simulink library "autolibbatterycommon"  (R2019b)
settings: Solver=ode45  StartTime=0.0  StopTime=10.0  RelTol=1e-3  EnableMultiTasking=on
undefined symbols (not defined in the file or in its folder): BattCap, BattCapInit, BattChargeMax, BattTempBp, C, C1, C2, C3, C4, C5, Cap_LUT, CapacityAh, CapLUTBp, CapSOCBp, CapVolt, Current_BP, DiscIntNeverNeededParam, Em, InitialCapVoltage, InitialChargeRemAh, Np, Ns, R, R0, R1, R2, R3, R4, R5, RefBlkName, RInt, SOC_BP, T1, Tc, Temp_BP, Temperature_BP, Ts, Vinit, Vu
libraries: $bdroot x72, autolibpowerinfoutils x1
(part 1 of 2)
settings Model: ModifiedByFormat=The MathWorks, Inc.  Creator=The MathWorks, Inc.  LastModifiedBy=The MathWorks, Inc.
settings DataIOCC: LimitDataPoints=on  SaveFormat=Array  ReturnWorkspaceOutputs=off
settings OptimizationCC: LifeSpan=inf
settings DebuggingCC: AllowSymbolicDim=off  PregeneratedLibrarySubsystemCodeDiagnostic=none  SFUnexpectedBacktrackingDiag=warning  SFNoUnconditionalDefaultTransitionDiag=warning  SFExecutionAtInitializationDiag=none  ArithmeticOperatorsInVariantConditions=warning
settings HardwareCC: ProdBitPerPointer=32  ProdBitPerSizeT=32  ProdBitPerPtrDiffT=32  ProdLargestAtomicFloat=None  ProdIntDivRoundTo=Undefined  ProdEndianess=Unspecified  ProdWordSize=32  ProdHWDeviceType=32-bit Generic
settings ModelReferenceCC: PropagateSignalLabelsOutOfModel=off
settings SFSimCC: SimUseLocalCustomCode=off  CustomCodeUndefinedFunction=UseInterfaceOnly
settings RTWCC: RTWUseLocalCustomCode=off
settings CodeAppCC: StateflowObjectComments=on
settings GRTTargetCC: TargetLangStandard=C89/C90 (ANSI)  GeneratePreprocessorConditionals=Disable all
settings ConfigComp: CovMetricSettings=dw  CovHtmlReporting=on  CovSaveCumulativeToWorkspaceVar=on  CovSaveSingleToWorkspaceVar=on  CovShowResultsExplorer=off  CovExternalEMLEnable=off

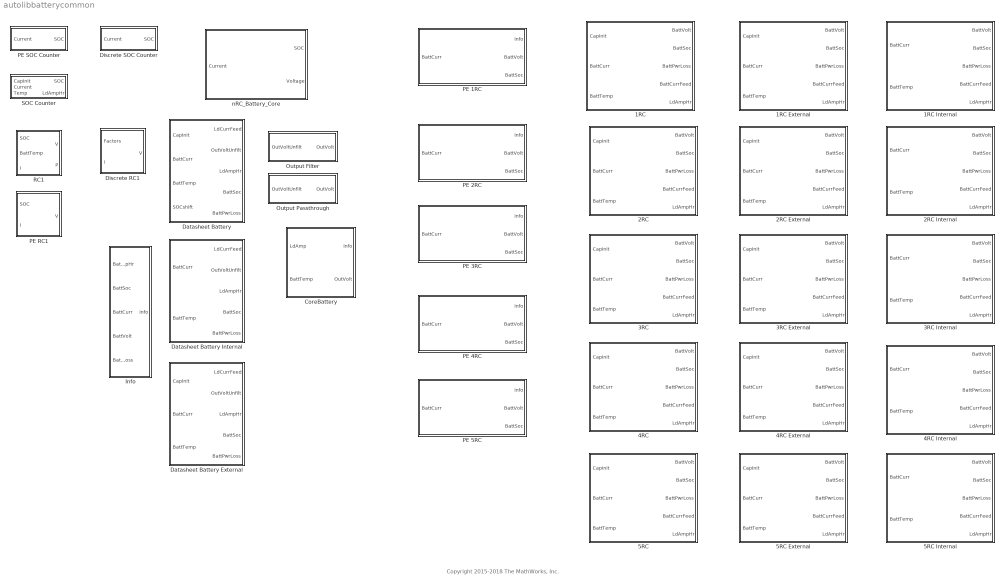
== system autolibbatterycommon ==
  note: Copyright 2015-2018 The MathWorks, Inc.
  1RC : Subsystem  VariantControl=1
  1RC External : Subsystem
  1RC Internal : Subsystem
  2RC : Subsystem  VariantControl=1
  2RC External : Subsystem
  2RC Internal : Subsystem
  3RC : Subsystem  VariantControl=1
  3RC External : Subsystem
  3RC Internal : Subsystem
  4RC : Subsystem  VariantControl=1
  4RC External : Subsystem
  4RC Internal : Subsystem
  5RC : Subsystem  VariantControl=1
  5RC External : Subsystem
  5RC Internal : Subsystem
  CoreBattery : Subsystem
  Datasheet Battery : Subsystem
  Datasheet Battery External : Subsystem
  Datasheet Battery Internal : Subsystem
  Discrete RC1 : Subsystem  mask(RCBlock){R=R1, Tau=T1, SOC_LUT=SOC_BP, Current_BP=Current_BP, V_init=InitialCapVoltage(1), V_upper=Vu(1), V_lower=Vu(1), T=Ts}
      mask prompts: R "Parallel Resistance Lookup Table"; Tau "Parallel Time Constant Lookup Table"; SOC_LUT "SOC Breakpoints"; Current_BP "Current Breakpoints"; V_init "Initial Voltage Across Capacitor"; V_upper "Upper Integrator Voltage Limit"; V_lower "Lower Integrator Voltage Limit"; T "Sample Time"
      mask help: Models a resistor and capacitor in parallel. Both components may vary with SOC.
  Discrete SOC Counter : Subsystem  mask(AhCounter){Q_init=InitialChargeRemAh, Cap=CapacityAh, T=Ts}
      mask prompts: Q_init "Initial Charge (Q)"; Cap "Capacity (Ah)"; T "Sample Time (s)"
      mask help: This is a system that keeps track of SOC by counting coulombs.
  Info : Subsystem  mask{RefBlkName=RefBlkName}
      mask prompts: RefBlkName "Reference block name:"
      mask TypeOptions RefBlkName: Power Accounting Bus Creator/RefBlkName
  Output Filter : Subsystem
  Output Passthrough : Subsystem
  PE 1RC : Subsystem  VariantControl=1
  PE 2RC : Subsystem  VariantControl=2
  PE 3RC : Subsystem  VariantControl=3
  PE 4RC : Subsystem  VariantControl=4
  PE 5RC : Subsystem  VariantControl=5
  PE RC1 : Subsystem  mask(RCBlock){R=R, C=C, SOC_BP=SOC_BP, V_init=CapVolt, V_upper=Inf, V_lower=-Inf}
      mask prompts: R "Parallel Resistance Lookup Table"; C "Parallel Capacitance Lookup Table"; SOC_BP "SOC Breakpoints"; V_init "Initial Voltage Across Capacitor"; V_upper "Upper Integrator Voltage Limit"; V_lower "Lower Integrator Voltage Limit"
      mask help: Models a resistor and capacitor in parallel. Both components may vary with SOC.
  PE SOC Counter : Subsystem  mask(AhCounter){Q_init=BattCapInit, Cap=BattCap}
      mask prompts: Q_init "Initial Charge"; Cap "Capacity"
      mask help: This is a system that keeps track of SOC by counting coulombs.
  RC1 : Subsystem  mask(RCBlock){R=R, C=C, SOC_BP=SOC_BP, Temperature_BP=Temp_BP, V_init=CapVolt, V_upper=Inf, V_lower=-Inf}
      mask prompts: R "Parallel Resistance Lookup Table"; C "Parallel Capacitance Lookup Table"; SOC_BP "SOC Breakpoints"; Temperature_BP "Temperature Breakpoints"; V_init "Initial Voltage Across Capacitor"; V_upper "Upper Integrator Voltage Limit"; V_lower "Lower Integrator Voltage Limit"
      mask help: Models a resistor and capacitor in parallel. Both components may vary with SOC.
  SOC Counter : Subsystem  mask(AhCounter){Q_init=BattCapInit, Cap=BattCap, Cap_LUT=Cap_LUT, Temp_BP=Temperature_BP}
      mask prompts: Q_init "Initial Charge"; Cap "Capacity"; Cap_LUT "Capacity temperature table"; Temp_BP "Temperature Break Points"
      mask help: This is a system that keeps track of SOC by counting coulombs.
  nRC_Battery_Core : Subsystem  VariantControlMode=Label  Variant=on  LabelModeActiveChoice=3

== system autolibbatterycommon/1RC ==
  CapInit : Inport  Unit=A*hr
  BattCurr : Inport  Port=2  Unit=A
  BattTemp : Inport  Port=3  Unit=K
  Em : Lookup_n-D  LookupTableObject=''  BreakpointsForDimension1=SOC_BP  BreakpointsForDimension2=Temperature_BP  Table=Em  ExtrapMethod=Clip  UseLastTableValue=on  InternalRulePriority=Speed  RndMeth=Simplest  InputSameDT=on
  Power : Subsystem
  R0 : Lookup_n-D  LookupTableObject=''  BreakpointsForDimension1=SOC_BP  BreakpointsForDimension2=Temperature_BP  Table=R0  ExtrapMethod=Clip  UseLastTableValue=on  InternalRulePriority=Speed  RndMeth=Simplest  InputSameDT=on
  RC1 : $bdroot/RC1  R=R1  C=C1  SOC_BP=SOC_BP  Temperature_BP=Temperature_BP  V_init=InitialCapVoltage(1)  V_upper=Vu  V_lower=Vl
  SOC Counter : $bdroot/SOC Counter  Q_init=BattCapInit  Cap=BattCap  Cap_LUT=BattCap  Temp_BP=Temperature_BP
  Voltage : Subsystem
  BattVolt : Outport  Unit=V  VectorParamsAs1DForOutWhenUnconnected=off
  BattSoc : Outport  Port=2  Unit=1  VectorParamsAs1DForOutWhenUnconnected=off
  BattPwrLoss : Outport  Port=3  Unit=W  VectorParamsAs1DForOutWhenUnconnected=off
  BattCurrFeed : Outport  Port=4  Unit=A  VectorParamsAs1DForOutWhenUnconnected=off
  LdAmpHr : Outport  Port=5  Unit=A*h  VectorParamsAs1DForOutWhenUnconnected=off
  wires:
  SOC Counter/1 -> R0/1, RC1/1, Em/1, BattSoc/1
  BattCurr/1 -> SOC Counter/2, Power/2(BattAmp), Voltage/3(BattAmp), BattCurrFeed/1, RC1/3
  BattTemp/1 -> SOC Counter/3, RC1/2, R0/2, Em/2
  Em/1 -> Voltage/1(Em)
  R0/1 -> Power/1(R0), Voltage/2(R0)
  RC1/1 -> Voltage/4(RC1)
  Voltage/1(BattVolt) -> BattVolt/1
  Power/1(BattPwrLoss) -> BattPwrLoss/1
  RC1/2 -> Power/3(P1)
  CapInit/1 -> SOC Counter/1
  SOC Counter/2 -> LdAmpHr/1

== system autolibbatterycommon/1RC External ==
  CapInit : Inport
  BattCurr : Inport  Port=2
  BattTemp : Inport  Port=3
  1RC : $bdroot/1RC  SystemSampleTime=-1  VariantControl=1  Latency=0  AutoFrameSizeCalculation=off
  BattVolt : Outport  VectorParamsAs1DForOutWhenUnconnected=off
  BattSoc : Outport  Port=2  VectorParamsAs1DForOutWhenUnconnected=off
  BattPwrLoss : Outport  Port=3  VectorParamsAs1DForOutWhenUnconnected=off
  BattCurrFeed : Outport  Port=4  VectorParamsAs1DForOutWhenUnconnected=off
  LdAmpHr : Outport  Port=5  VectorParamsAs1DForOutWhenUnconnected=off
  wires:
  BattCurr/1 -> 1RC/2
  BattTemp/1 -> 1RC/3
  1RC/1 -> BattVolt/1
  1RC/2 -> BattSoc/1
  1RC/3 -> BattPwrLoss/1
  1RC/4 -> BattCurrFeed/1
  CapInit/1 -> 1RC/1
  1RC/5 -> LdAmpHr/1

== system autolibbatterycommon/1RC Internal ==
  BattCurr : Inport
  BattTemp : Inport  Port=2
  1RC : $bdroot/1RC  SystemSampleTime=-1  VariantControl=1  Latency=0  AutoFrameSizeCalculation=off
  Constant1 : Constant  Value=BattCapInit
  BattVolt : Outport  VectorParamsAs1DForOutWhenUnconnected=off
  BattSoc : Outport  Port=2  VectorParamsAs1DForOutWhenUnconnected=off
  BattPwrLoss : Outport  Port=3  VectorParamsAs1DForOutWhenUnconnected=off
  BattCurrFeed : Outport  Port=4  VectorParamsAs1DForOutWhenUnconnected=off
  LdAmpHr : Outport  Port=5  VectorParamsAs1DForOutWhenUnconnected=off
  wires:
  BattCurr/1 -> 1RC/2
  BattTemp/1 -> 1RC/3
  1RC/1 -> BattVolt/1
  1RC/2 -> BattSoc/1
  1RC/3 -> BattPwrLoss/1
  1RC/4 -> BattCurrFeed/1
  Constant1/1 -> 1RC/1
  1RC/5 -> LdAmpHr/1

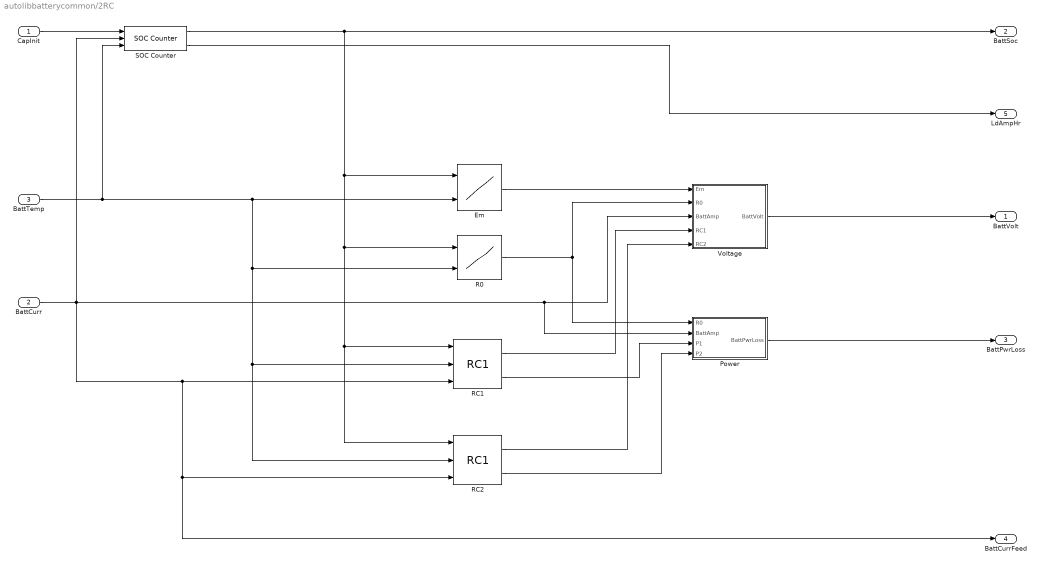
== system autolibbatterycommon/2RC ==
  CapInit : Inport  Unit=A*hr
  BattCurr : Inport  Port=2  Unit=A
  BattTemp : Inport  Port=3  Unit=K
  Em : Lookup_n-D  LookupTableObject=''  BreakpointsForDimension1=SOC_BP  BreakpointsForDimension2=Temperature_BP  Table=Em  ExtrapMethod=Clip  UseLastTableValue=on  InternalRulePriority=Speed  RndMeth=Simplest  InputSameDT=on
  Power : Subsystem
  R0 : Lookup_n-D  LookupTableObject=''  BreakpointsForDimension1=SOC_BP  BreakpointsForDimension2=Temperature_BP  Table=R0  ExtrapMethod=Clip  UseLastTableValue=on  InternalRulePriority=Speed  RndMeth=Simplest  InputSameDT=on
  RC1 : $bdroot/RC1  R=R1  C=C1  SOC_BP=SOC_BP  Temperature_BP=Temperature_BP  V_init=InitialCapVoltage(1)  V_upper=Vu  V_lower=Vl
  RC2 : $bdroot/RC1  R=R2  C=C2  SOC_BP=SOC_BP  Temperature_BP=Temperature_BP  V_init=InitialCapVoltage(2)  V_upper=Vu  V_lower=Vl
  SOC Counter : $bdroot/SOC Counter  Q_init=BattCapInit  Cap=BattCap  Cap_LUT=BattCap  Temp_BP=Temperature_BP
  Voltage : Subsystem
  BattVolt : Outport  Unit=V  VectorParamsAs1DForOutWhenUnconnected=off
  BattSoc : Outport  Port=2  Unit=1  VectorParamsAs1DForOutWhenUnconnected=off
  BattPwrLoss : Outport  Port=3  Unit=W  VectorParamsAs1DForOutWhenUnconnected=off
  BattCurrFeed : Outport  Port=4  Unit=A  VectorParamsAs1DForOutWhenUnconnected=off
  LdAmpHr : Outport  Port=5  Unit=A*h  VectorParamsAs1DForOutWhenUnconnected=off
  wires:
  SOC Counter/1 -> R0/1, RC2/1, RC1/1, Em/1, BattSoc/1
  BattCurr/1 -> SOC Counter/2, Power/2(BattAmp), Voltage/3(BattAmp), BattCurrFeed/1, RC2/3, RC1/3
  BattTemp/1 -> SOC Counter/3, RC2/2, RC1/2, R0/2, Em/2
  Em/1 -> Voltage/1(Em)
  R0/1 -> Power/1(R0), Voltage/2(R0)
  RC1/1 -> Voltage/4(RC1)
  RC2/1 -> Voltage/5(RC2)
  Voltage/1(BattVolt) -> BattVolt/1
  RC1/2 -> Power/3(P1)
  RC2/2 -> Power/4(P2)
  Power/1(BattPwrLoss) -> BattPwrLoss/1
  CapInit/1 -> SOC Counter/1
  SOC Counter/2 -> LdAmpHr/1

== system autolibbatterycommon/2RC External ==
  CapInit : Inport
  BattCurr : Inport  Port=2
  BattTemp : Inport  Port=3
  2RC : $bdroot/2RC  SystemSampleTime=-1  VariantControl=1  Latency=0  AutoFrameSizeCalculation=off
  BattVolt : Outport  VectorParamsAs1DForOutWhenUnconnected=off
  BattSoc : Outport  Port=2  VectorParamsAs1DForOutWhenUnconnected=off
  BattPwrLoss : Outport  Port=3  VectorParamsAs1DForOutWhenUnconnected=off
  BattCurrFeed : Outport  Port=4  VectorParamsAs1DForOutWhenUnconnected=off
  LdAmpHr : Outport  Port=5  VectorParamsAs1DForOutWhenUnconnected=off
  wires:
  BattTemp/1 -> 2RC/3
  BattCurr/1 -> 2RC/2
  CapInit/1 -> 2RC/1
  2RC/1 -> BattVolt/1
  2RC/2 -> BattSoc/1
  2RC/3 -> BattPwrLoss/1
  2RC/4 -> BattCurrFeed/1
  2RC/5 -> LdAmpHr/1

== system autolibbatterycommon/2RC Internal ==
  BattCurr : Inport
  BattTemp : Inport  Port=2
  2RC : $bdroot/2RC  SystemSampleTime=-1  VariantControl=1  Latency=0  AutoFrameSizeCalculation=off
  Constant1 : Constant  Value=BattCapInit
  BattVolt : Outport  VectorParamsAs1DForOutWhenUnconnected=off
  BattSoc : Outport  Port=2  VectorParamsAs1DForOutWhenUnconnected=off
  BattPwrLoss : Outport  Port=3  VectorParamsAs1DForOutWhenUnconnected=off
  BattCurrFeed : Outport  Port=4  VectorParamsAs1DForOutWhenUnconnected=off
  LdAmpHr : Outport  Port=5  VectorParamsAs1DForOutWhenUnconnected=off
  wires:
  BattTemp/1 -> 2RC/3
  BattCurr/1 -> 2RC/2
  2RC/1 -> BattVolt/1
  2RC/2 -> BattSoc/1
  2RC/3 -> BattPwrLoss/1
  2RC/4 -> BattCurrFeed/1
  Constant1/1 -> 2RC/1
  2RC/5 -> LdAmpHr/1

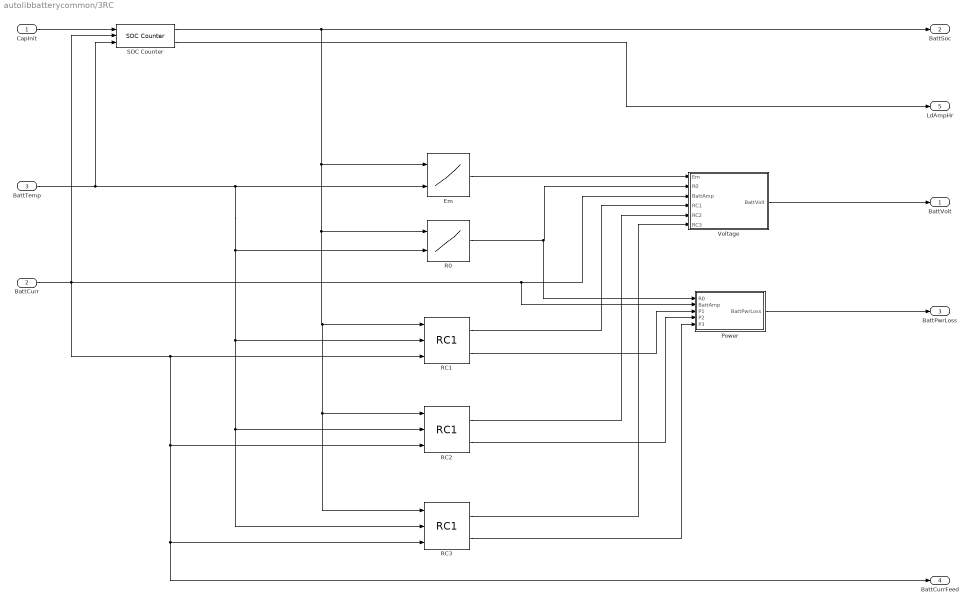
== system autolibbatterycommon/3RC ==
  CapInit : Inport  Unit=A*hr
  BattCurr : Inport  Port=2  Unit=A
  BattTemp : Inport  Port=3  Unit=K
  Em : Lookup_n-D  LookupTableObject=''  BreakpointsForDimension1=SOC_BP  BreakpointsForDimension2=Temperature_BP  Table=Em  ExtrapMethod=Clip  UseLastTableValue=on  InternalRulePriority=Speed  RndMeth=Simplest  InputSameDT=on
  Power : Subsystem
  R0 : Lookup_n-D  LookupTableObject=''  BreakpointsForDimension1=SOC_BP  BreakpointsForDimension2=Temperature_BP  Table=R0  ExtrapMethod=Clip  UseLastTableValue=on  InternalRulePriority=Speed  RndMeth=Simplest  InputSameDT=on
  RC1 : $bdroot/RC1  R=R1  C=C1  SOC_BP=SOC_BP  Temperature_BP=Temperature_BP  V_init=InitialCapVoltage(1)  V_upper=Vu  V_lower=Vl
  RC2 : $bdroot/RC1  R=R2  C=C2  SOC_BP=SOC_BP  Temperature_BP=Temperature_BP  V_init=InitialCapVoltage(2)  V_upper=Vu  V_lower=Vl
  RC3 : $bdroot/RC1  R=R3  C=C3  SOC_BP=SOC_BP  Temperature_BP=Temperature_BP  V_init=InitialCapVoltage(3)  V_upper=Vu  V_lower=Vl
  SOC Counter : $bdroot/SOC Counter  Q_init=BattCapInit  Cap=BattCap  Cap_LUT=BattCap  Temp_BP=Temperature_BP
  Voltage : Subsystem
  BattVolt : Outport  Unit=V  VectorParamsAs1DForOutWhenUnconnected=off
  BattSoc : Outport  Port=2  Unit=1  VectorParamsAs1DForOutWhenUnconnected=off
  BattPwrLoss : Outport  Port=3  Unit=W  VectorParamsAs1DForOutWhenUnconnected=off
  BattCurrFeed : Outport  Port=4  Unit=A  VectorParamsAs1DForOutWhenUnconnected=off
  LdAmpHr : Outport  Port=5  Unit=A*h  VectorParamsAs1DForOutWhenUnconnected=off
  wires:
  BattTemp/1 -> SOC Counter/3, Em/2, R0/2, RC1/2, RC3/2, RC2/2
  BattCurr/1 -> SOC Counter/2, Power/2(BattAmp), Voltage/3(BattAmp), RC1/3, RC2/3, BattCurrFeed/1, RC3/3
  SOC Counter/1 -> Em/1, RC1/1, RC3/1, RC2/1, R0/1, BattSoc/1
  Em/1 -> Voltage/1(Em)
  R0/1 -> Power/1(R0), Voltage/2(R0)
  RC1/1 -> Voltage/4(RC1)
  RC2/1 -> Voltage/5(RC2)
  RC3/1 -> Voltage/6(RC3)
  Voltage/1(BattVolt) -> BattVolt/1
  RC1/2 -> Power/3(P1)
  RC2/2 -> Power/4(P2)
  RC3/2 -> Power/5(P3)
  Power/1(BattPwrLoss) -> BattPwrLoss/1
  CapInit/1 -> SOC Counter/1
  SOC Counter/2 -> LdAmpHr/1

== system autolibbatterycommon/3RC External ==
  CapInit : Inport
  BattCurr : Inport  Port=2
  BattTemp : Inport  Port=3
  3RC : $bdroot/3RC  SystemSampleTime=-1  VariantControl=1  Latency=0  AutoFrameSizeCalculation=off
  BattVolt : Outport  VectorParamsAs1DForOutWhenUnconnected=off
  BattSoc : Outport  Port=2  VectorParamsAs1DForOutWhenUnconnected=off
  BattPwrLoss : Outport  Port=3  VectorParamsAs1DForOutWhenUnconnected=off
  BattCurrFeed : Outport  Port=4  VectorParamsAs1DForOutWhenUnconnected=off
  LdAmpHr : Outport  Port=5  VectorParamsAs1DForOutWhenUnconnected=off
  wires:
  3RC/4 -> BattCurrFeed/1
  3RC/2 -> BattSoc/1
  3RC/1 -> BattVolt/1
  3RC/3 -> BattPwrLoss/1
  BattTemp/1 -> 3RC/3
  BattCurr/1 -> 3RC/2
  CapInit/1 -> 3RC/1
  3RC/5 -> LdAmpHr/1

== system autolibbatterycommon/3RC Internal ==
  BattCurr : Inport
  BattTemp : Inport  Port=2
  3RC : $bdroot/3RC  SystemSampleTime=-1  VariantControl=1  Latency=0  AutoFrameSizeCalculation=off
  Constant1 : Constant  Value=BattCapInit
  BattVolt : Outport  VectorParamsAs1DForOutWhenUnconnected=off
  BattSoc : Outport  Port=2  VectorParamsAs1DForOutWhenUnconnected=off
  BattPwrLoss : Outport  Port=3  VectorParamsAs1DForOutWhenUnconnected=off
  BattCurrFeed : Outport  Port=4  VectorParamsAs1DForOutWhenUnconnected=off
  LdAmpHr : Outport  Port=5  VectorParamsAs1DForOutWhenUnconnected=off
  wires:
  3RC/4 -> BattCurrFeed/1
  3RC/2 -> BattSoc/1
  3RC/1 -> BattVolt/1
  3RC/3 -> BattPwrLoss/1
  BattTemp/1 -> 3RC/3
  BattCurr/1 -> 3RC/2
  Constant1/1 -> 3RC/1
  3RC/5 -> LdAmpHr/1

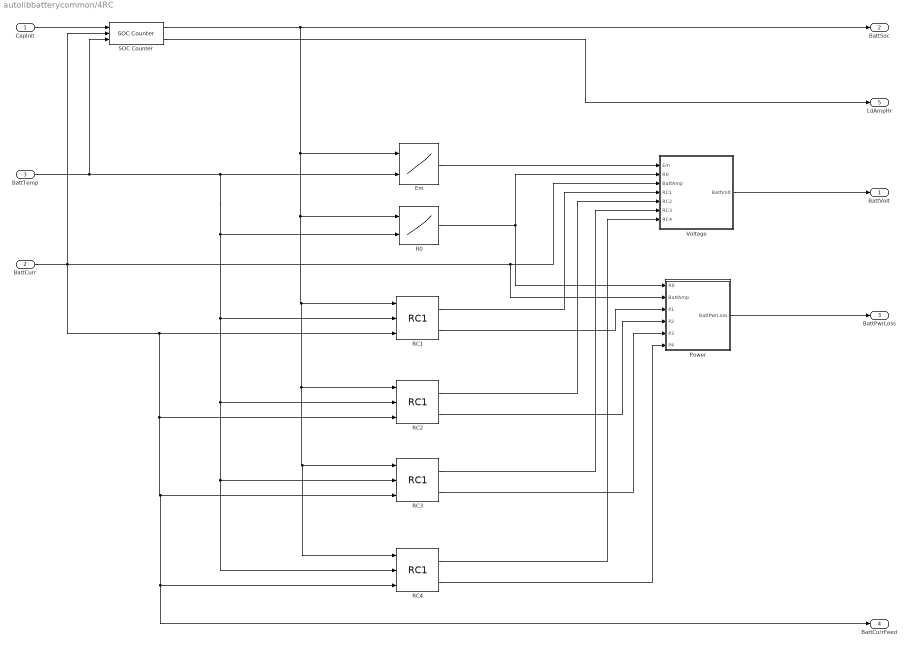
== system autolibbatterycommon/4RC ==
  CapInit : Inport  Unit=A*hr
  BattCurr : Inport  Port=2  Unit=A
  BattTemp : Inport  Port=3  Unit=K
  Em : Lookup_n-D  LookupTableObject=''  BreakpointsForDimension1=SOC_BP  BreakpointsForDimension2=Temperature_BP  Table=Em  ExtrapMethod=Clip  UseLastTableValue=on  InternalRulePriority=Speed  RndMeth=Simplest  InputSameDT=on
  Power : Subsystem
  R0 : Lookup_n-D  LookupTableObject=''  BreakpointsForDimension1=SOC_BP  BreakpointsForDimension2=Temperature_BP  Table=R0  ExtrapMethod=Clip  UseLastTableValue=on  InternalRulePriority=Speed  RndMeth=Simplest  InputSameDT=on
  RC1 : $bdroot/RC1  R=R1  C=C1  SOC_BP=SOC_BP  Temperature_BP=Temperature_BP  V_init=InitialCapVoltage(1)  V_upper=Vu  V_lower=Vl
  RC2 : $bdroot/RC1  R=R2  C=C2  SOC_BP=SOC_BP  Temperature_BP=Temperature_BP  V_init=InitialCapVoltage(2)  V_upper=Vu  V_lower=Vl
  RC3 : $bdroot/RC1  R=R3  C=C3  SOC_BP=SOC_BP  Temperature_BP=Temperature_BP  V_init=InitialCapVoltage(3)  V_upper=Vu  V_lower=Vl
  RC4 : $bdroot/RC1  R=R4  C=C4  SOC_BP=SOC_BP  Temperature_BP=Temperature_BP  V_init=InitialCapVoltage(4)  V_upper=Vu  V_lower=Vl
  SOC Counter : $bdroot/SOC Counter  Q_init=BattCapInit  Cap=BattCap  Cap_LUT=BattCap  Temp_BP=Temperature_BP
  Voltage : Subsystem
  BattVolt : Outport  Unit=V  VectorParamsAs1DForOutWhenUnconnected=off
  BattSoc : Outport  Port=2  Unit=1  VectorParamsAs1DForOutWhenUnconnected=off
  BattPwrLoss : Outport  Port=3  Unit=W  VectorParamsAs1DForOutWhenUnconnected=off
  BattCurrFeed : Outport  Port=4  Unit=A  VectorParamsAs1DForOutWhenUnconnected=off
  LdAmpHr : Outport  Port=5  Unit=A*h  VectorParamsAs1DForOutWhenUnconnected=off
  wires:
  SOC Counter/1 -> R0/1, RC2/1, RC4/1, RC3/1, RC1/1, Em/1, BattSoc/1
  BattCurr/1 -> SOC Counter/2, Power/2(BattAmp), Voltage/3(BattAmp), RC4/3, BattCurrFeed/1, RC3/3, RC2/3, RC1/3
  BattTemp/1 -> SOC Counter/3, RC2/2, RC4/2, RC3/2, RC1/2, R0/2, Em/2
  Em/1 -> Voltage/1(Em)
  R0/1 -> Power/1(R0), Voltage/2(R0)
  RC1/1 -> Voltage/4(RC1)
  RC2/1 -> Voltage/5(RC2)
  RC3/1 -> Voltage/6(RC3)
  RC4/1 -> Voltage/7(RC4)
  Voltage/1(BattVolt) -> BattVolt/1
  Power/1(BattPwrLoss) -> BattPwrLoss/1
  RC1/2 -> Power/3(P1)
  RC2/2 -> Power/4(P2)
  RC3/2 -> Power/5(P3)
  RC4/2 -> Power/6(P4)
  CapInit/1 -> SOC Counter/1
  SOC Counter/2 -> LdAmpHr/1

== system autolibbatterycommon/4RC External ==
  CapInit : Inport
  BattCurr : Inport  Port=2
  BattTemp : Inport  Port=3
  4RC : $bdroot/4RC  SystemSampleTime=-1  VariantControl=1  Latency=0  AutoFrameSizeCalculation=off
  BattVolt : Outport  VectorParamsAs1DForOutWhenUnconnected=off
  BattSoc : Outport  Port=2  VectorParamsAs1DForOutWhenUnconnected=off
  BattPwrLoss : Outport  Port=3  VectorParamsAs1DForOutWhenUnconnected=off
  BattCurrFeed : Outport  Port=4  VectorParamsAs1DForOutWhenUnconnected=off
  LdAmpHr : Outport  Port=5  VectorParamsAs1DForOutWhenUnconnected=off
  wires:
  BattTemp/1 -> 4RC/3
  BattCurr/1 -> 4RC/2
  CapInit/1 -> 4RC/1
  4RC/1 -> BattVolt/1
  4RC/2 -> BattSoc/1
  4RC/3 -> BattPwrLoss/1
  4RC/4 -> BattCurrFeed/1
  4RC/5 -> LdAmpHr/1

== system autolibbatterycommon/4RC Internal ==
  BattCurr : Inport
  BattTemp : Inport  Port=2
  4RC : $bdroot/4RC  SystemSampleTime=-1  VariantControl=1  Latency=0  AutoFrameSizeCalculation=off
  Constant1 : Constant  Value=BattCapInit
  BattVolt : Outport  VectorParamsAs1DForOutWhenUnconnected=off
  BattSoc : Outport  Port=2  VectorParamsAs1DForOutWhenUnconnected=off
  BattPwrLoss : Outport  Port=3  VectorParamsAs1DForOutWhenUnconnected=off
  BattCurrFeed : Outport  Port=4  VectorParamsAs1DForOutWhenUnconnected=off
  LdAmpHr : Outport  Port=5  VectorParamsAs1DForOutWhenUnconnected=off
  wires:
  BattTemp/1 -> 4RC/3
  BattCurr/1 -> 4RC/2
  4RC/1 -> BattVolt/1
  4RC/2 -> BattSoc/1
  4RC/3 -> BattPwrLoss/1
  4RC/4 -> BattCurrFeed/1
  Constant1/1 -> 4RC/1
  4RC/5 -> LdAmpHr/1

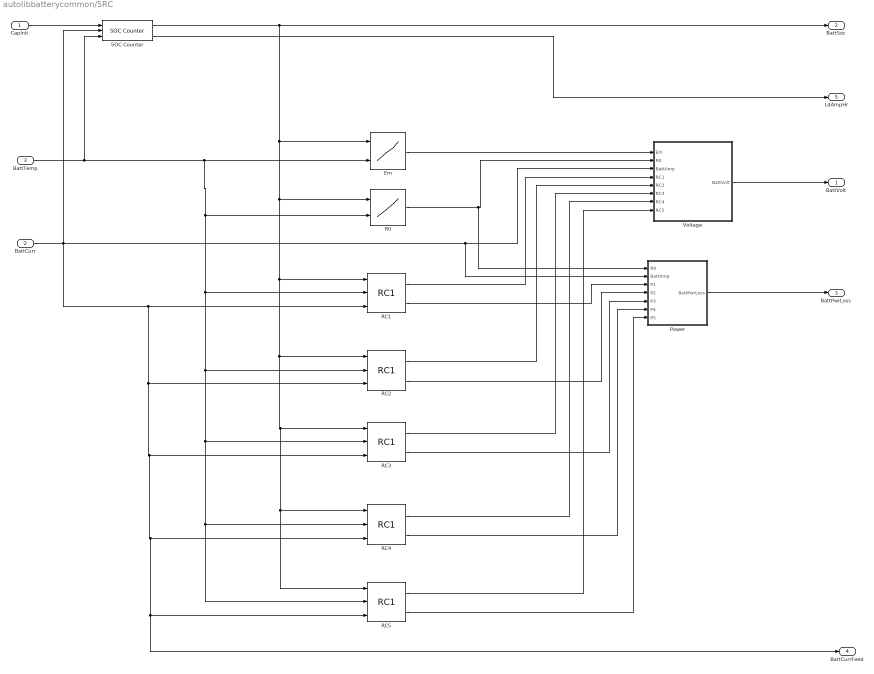
== system autolibbatterycommon/5RC ==
  CapInit : Inport  Unit=A*hr
  BattCurr : Inport  Port=2  Unit=A
  BattTemp : Inport  Port=3  Unit=K
  Em : Lookup_n-D  LookupTableObject=''  BreakpointsForDimension1=SOC_BP  BreakpointsForDimension2=Temperature_BP  Table=Em  ExtrapMethod=Clip  UseLastTableValue=on  InternalRulePriority=Speed  RndMeth=Simplest  InputSameDT=on
  Power : Subsystem
  R0 : Lookup_n-D  LookupTableObject=''  BreakpointsForDimension1=SOC_BP  BreakpointsForDimension2=Temperature_BP  Table=R0  ExtrapMethod=Clip  UseLastTableValue=on  InternalRulePriority=Speed  RndMeth=Simplest  InputSameDT=on
  RC1 : $bdroot/RC1  R=R1  C=C1  SOC_BP=SOC_BP  Temperature_BP=Temperature_BP  V_init=InitialCapVoltage(1)  V_upper=Vu  V_lower=Vl
  RC2 : $bdroot/RC1  R=R2  C=C2  SOC_BP=SOC_BP  Temperature_BP=Temperature_BP  V_init=InitialCapVoltage(2)  V_upper=Vu  V_lower=Vl
  RC3 : $bdroot/RC1  R=R3  C=C3  SOC_BP=SOC_BP  Temperature_BP=Temperature_BP  V_init=InitialCapVoltage(3)  V_upper=Vu  V_lower=Vl
  RC4 : $bdroot/RC1  R=R4  C=C4  SOC_BP=SOC_BP  Temperature_BP=Temperature_BP  V_init=InitialCapVoltage(4)  V_upper=Vu  V_lower=Vl
  RC5 : $bdroot/RC1  R=R5  C=C5  SOC_BP=SOC_BP  Temperature_BP=Temperature_BP  V_init=InitialCapVoltage(5)  V_upper=Vu  V_lower=Vl
  SOC Counter : $bdroot/SOC Counter  Q_init=BattCapInit  Cap=BattCap  Cap_LUT=BattCap  Temp_BP=Temperature_BP
  Voltage : Subsystem
  BattVolt : Outport  Unit=V  VectorParamsAs1DForOutWhenUnconnected=off
  BattSoc : Outport  Port=2  Unit=1  VectorParamsAs1DForOutWhenUnconnected=off
  BattPwrLoss : Outport  Port=3  Unit=W  VectorParamsAs1DForOutWhenUnconnected=off
  BattCurrFeed : Outport  Port=4  Unit=A  VectorParamsAs1DForOutWhenUnconnected=off
  LdAmpHr : Outport  Port=5  Unit=A*h  VectorParamsAs1DForOutWhenUnconnected=off
  wires:
  BattTemp/1 -> SOC Counter/3, Em/2, R0/2, RC1/2, RC3/2, RC5/2, RC4/2, RC2/2
  BattCurr/1 -> SOC Counter/2, Power/2(BattAmp), Voltage/3(BattAmp), RC1/3, RC2/3, RC3/3, BattCurrFeed/1, RC5/3, RC4/3
  SOC Counter/1 -> Em/1, RC1/1, RC3/1, RC5/1, RC4/1, RC2/1, R0/1, BattSoc/1
  Em/1 -> Voltage/1(Em)
  R0/1 -> Power/1(R0), Voltage/2(R0)
  RC1/1 -> Voltage/4(RC1)
  RC2/1 -> Voltage/5(RC2)
  RC3/1 -> Voltage/6(RC3)
  RC4/1 -> Voltage/7(RC4)
  RC5/1 -> Voltage/8(RC5)
  Voltage/1(BattVolt) -> BattVolt/1
  RC1/2 -> Power/3(P1)
  RC2/2 -> Power/4(P2)
  RC3/2 -> Power/5(P3)
  RC4/2 -> Power/6(P4)
  RC5/2 -> Power/7(P5)
  Power/1(BattPwrLoss) -> BattPwrLoss/1
  CapInit/1 -> SOC Counter/1
  SOC Counter/2 -> LdAmpHr/1

== system autolibbatterycommon/5RC External ==
  CapInit : Inport
  BattCurr : Inport  Port=2
  BattTemp : Inport  Port=3
  5RC : $bdroot/5RC  SystemSampleTime=-1  VariantControl=1  Latency=0  AutoFrameSizeCalculation=off
  BattVolt : Outport  VectorParamsAs1DForOutWhenUnconnected=off
  BattSoc : Outport  Port=2  VectorParamsAs1DForOutWhenUnconnected=off
  BattPwrLoss : Outport  Port=3  VectorParamsAs1DForOutWhenUnconnected=off
  BattCurrFeed : Outport  Port=4  VectorParamsAs1DForOutWhenUnconnected=off
  LdAmpHr : Outport  Port=5  VectorParamsAs1DForOutWhenUnconnected=off
  wires:
  BattTemp/1 -> 5RC/3
  BattCurr/1 -> 5RC/2
  CapInit/1 -> 5RC/1
  5RC/1 -> BattVolt/1
  5RC/2 -> BattSoc/1
  5RC/3 -> BattPwrLoss/1
  5RC/4 -> BattCurrFeed/1
  5RC/5 -> LdAmpHr/1

== system autolibbatterycommon/5RC Internal ==
  BattCurr : Inport
  BattTemp : Inport  Port=2
  5RC : $bdroot/5RC  SystemSampleTime=-1  VariantControl=1  Latency=0  AutoFrameSizeCalculation=off
  Constant1 : Constant  Value=BattCapInit
  BattVolt : Outport  VectorParamsAs1DForOutWhenUnconnected=off
  BattSoc : Outport  Port=2  VectorParamsAs1DForOutWhenUnconnected=off
  BattPwrLoss : Outport  Port=3  VectorParamsAs1DForOutWhenUnconnected=off
  BattCurrFeed : Outport  Port=4  VectorParamsAs1DForOutWhenUnconnected=off
  LdAmpHr : Outport  Port=5  VectorParamsAs1DForOutWhenUnconnected=off
  wires:
  BattTemp/1 -> 5RC/3
  BattCurr/1 -> 5RC/2
  5RC/1 -> BattVolt/1
  5RC/2 -> BattSoc/1
  5RC/3 -> BattPwrLoss/1
  5RC/4 -> BattCurrFeed/1
  Constant1/1 -> 5RC/1
  5RC/5 -> LdAmpHr/1

== system autolibbatterycommon/CoreBattery ==
  note: Info
  LdAmp : Inport
  BattTemp : Inport  Port=2
  Bus Creator : BusCreator  Inputs=4
  Charge Model : Subsystem
  State of Charge Capacity : Subsystem
  Subsystem : Subsystem
  Info : Outport  VectorParamsAs1DForOutWhenUnconnected=off
  OutVolt : Outport  Port=2  VectorParamsAs1DForOutWhenUnconnected=off
  wires:
  Subsystem/1(OutVolt) -> OutVolt/1, Bus Creator/4  "OutVolt"
  BattTemp/1 -> Subsystem/3(BattTemp)
  Charge Model/1(LdAmpHr) -> State of Charge Capacity/1(LdAmpHr), Bus Creator/2  "LdAmpHr"
  Bus Creator/1 -> Info/1
  LdAmp/1 -> Charge Model/1(LdAmp), Bus Creator/1, Subsystem/2(LdAmp)  "LdAmp"
  State of Charge Capacity/1(CapSOC) -> Subsystem/1(CapSOC), Bus Creator/3  "CapSOC"

== system autolibbatterycommon/Datasheet Battery ==
  CapInit : Inport  Unit=A*hr
  BattCurr : Inport  Port=2  Unit=A
  BattTemp : Inport  Port=3  Unit=K
  SOCshift : Inport  Port=4  Unit=1
  Add : Sum
  Charge Model : Subsystem
  State of Charge Capacity : Subsystem
  Voltage and Power Calculation : Subsystem
  LdCurrFeed : Outport  Unit=A  VectorParamsAs1DForOutWhenUnconnected=off
  OutVoltUnfilt : Outport  Port=2  Unit=V  VectorParamsAs1DForOutWhenUnconnected=off
  LdAmpHr : Outport  Port=3  Unit=A*hr  VectorParamsAs1DForOutWhenUnconnected=off
  BattSoc : Outport  Port=4  Unit=1  VectorParamsAs1DForOutWhenUnconnected=off
  BattPwrLoss : Outport  Port=5  Unit=V  VectorParamsAs1DForOutWhenUnconnected=off
  wires:
  BattCurr/1 -> LdCurrFeed/1, Voltage and Power Calculation/2(LdAmp), Charge Model/1(LdAmp)
  Voltage and Power Calculation/1(OutVolt) -> OutVoltUnfilt/1
  Charge Model/1(LdAmpHr) -> State of Charge Capacity/1(LdAmpHr), LdAmpHr/1
  Add/1 -> Voltage and Power Calculation/1(CapSOC), BattSoc/1
  BattTemp/1 -> Voltage and Power Calculation/3(BattTemp)
  CapInit/1 -> Charge Model/2(CapInit)
  Voltage and Power Calculation/2(BattPwrLoss) -> BattPwrLoss/1
  State of Charge Capacity/1(CapSOC) -> Add/1
  SOCshift/1 -> Add/2

== system autolibbatterycommon/Datasheet Battery External ==
  CapInit : Inport
  BattCurr : Inport  Port=2
  BattTemp : Inport  Port=3
  Datasheet Battery : $bdroot/Datasheet Battery  SystemSampleTime=-1  Latency=0  AutoFrameSizeCalculation=off
  LdCurrFeed : Outport  VectorParamsAs1DForOutWhenUnconnected=off
  OutVoltUnfilt : Outport  Port=2  VectorParamsAs1DForOutWhenUnconnected=off
  LdAmpHr : Outport  Port=3  VectorParamsAs1DForOutWhenUnconnected=off
  BattSoc : Outport  Port=4  VectorParamsAs1DForOutWhenUnconnected=off
  BattPwrLoss : Outport  Port=5  VectorParamsAs1DForOutWhenUnconnected=off
  wires:
  BattTemp/1 -> Datasheet Battery/3
  BattCurr/1 -> Datasheet Battery/2
  CapInit/1 -> Datasheet Battery/1
  Datasheet Battery/4 -> BattSoc/1
  Datasheet Battery/3 -> LdAmpHr/1
  Datasheet Battery/2 -> OutVoltUnfilt/1
  Datasheet Battery/1 -> LdCurrFeed/1
  Datasheet Battery/5 -> BattPwrLoss/1

== system autolibbatterycommon/Datasheet Battery Internal ==
  BattCurr : Inport
  BattTemp : Inport  Port=2
  Constant1 : Constant  Value=BattCapInit
  Datasheet Battery : $bdroot/Datasheet Battery  SystemSampleTime=-1  Latency=0  AutoFrameSizeCalculation=off
  LdCurrFeed : Outport  VectorParamsAs1DForOutWhenUnconnected=off
  OutVoltUnfilt : Outport  Port=2  VectorParamsAs1DForOutWhenUnconnected=off
  LdAmpHr : Outport  Port=3  VectorParamsAs1DForOutWhenUnconnected=off
  BattSoc : Outport  Port=4  VectorParamsAs1DForOutWhenUnconnected=off
  BattPwrLoss : Outport  Port=5  VectorParamsAs1DForOutWhenUnconnected=off
  wires:
  Constant1/1 -> Datasheet Battery/1
  BattCurr/1 -> Datasheet Battery/2
  BattTemp/1 -> Datasheet Battery/3
  Datasheet Battery/4 -> BattSoc/1
  Datasheet Battery/3 -> LdAmpHr/1
  Datasheet Battery/2 -> OutVoltUnfilt/1
  Datasheet Battery/1 -> LdCurrFeed/1
  Datasheet Battery/5 -> BattPwrLoss/1

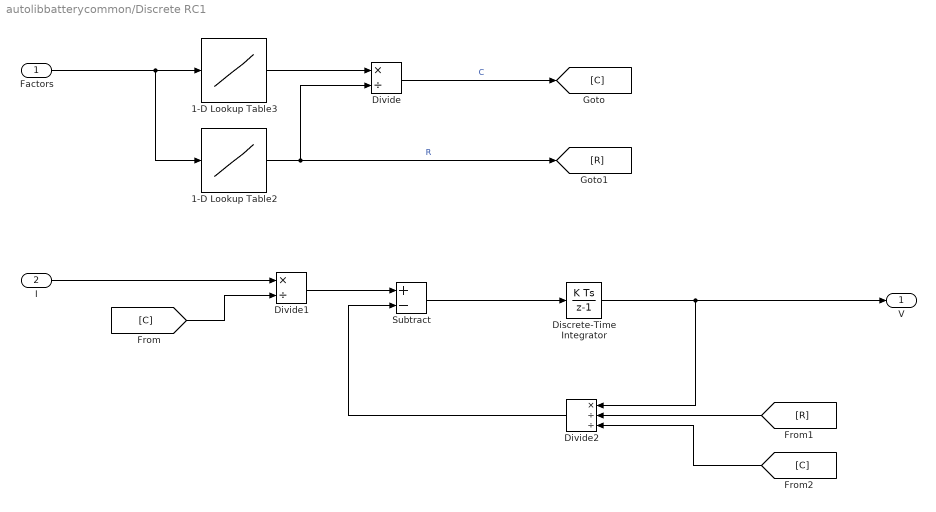
== system autolibbatterycommon/Discrete RC1 ==
  Factors : Inport
  I : Inport  Port=2
  1-D Lookup Table2 : Lookup_n-D  LookupTableObject=''  BreakpointsForDimension1=SOC_LUT  BreakpointsForDimension2=Current_BP  UseOneInputPortForAllInputData=on  Table=R  ExtrapMethod=Clip  UseLastTableValue=on  InternalRulePriority=Speed  RndMeth=Simplest  InputSameDT=on
  1-D Lookup Table3 : Lookup_n-D  LookupTableObject=''  BreakpointsForDimension1=SOC_LUT  BreakpointsForDimension2=Current_BP  UseOneInputPortForAllInputData=on  Table=Tau  ExtrapMethod=Clip  UseLastTableValue=on  InternalRulePriority=Speed  RndMeth=Simplest  InputSameDT=on
  Discrete-Time Integrator : DiscreteIntegrator  SampleTime=Ts  LimitOutput=on  UpperSaturationLimit=V_upper  LowerSaturationLimit=V_lower  ICPrevOutput=DiscIntNeverNeededParam  ICPrevScaledInput=DiscIntNeverNeededParam
  Divide : Product  Inputs=*/
  Divide1 : Product  Inputs=*/
  Divide2 : Product  Inputs=*//
  Subtract : Sum  Inputs=+-
  V : Outport  VectorParamsAs1DForOutWhenUnconnected=off
  wires:
  [C] -> Divide2/3
  [R] -> Divide2/2
  Divide2/1 -> Subtract/2
  [C] -> Divide1/2
  I/1 -> Divide1/1
  Divide/1 -> [C]  "C"
  1-D Lookup Table2/1 -> [R], Divide/2  "R"
  1-D Lookup Table3/1 -> Divide/1
  Factors/1 -> 1-D Lookup Table2/1, 1-D Lookup Table3/1
  Discrete-Time Integrator/1 -> V/1, Divide2/1
  Subtract/1 -> Discrete-Time Integrator/1
  Divide1/1 -> Subtract/1

== system autolibbatterycommon/Discrete SOC Counter ==
  Current : Inport
  Convert to Ah : Gain  Gain=1/3600
  Convert to SOC : Gain  Gain=1/Cap
  Discrete-Time Integrator : DiscreteIntegrator  InitialCondition=Q_init*3600  SampleTime=Ts  LimitOutput=on  UpperSaturationLimit=3600 * Cap  LowerSaturationLimit=0  ICPrevOutput=DiscIntNeverNeededParam  ICPrevScaledInput=DiscIntNeverNeededParam
  SOC : Outport  VectorParamsAs1DForOutWhenUnconnected=off
  wires:
  Discrete-Time Integrator/1 -> Convert to Ah/1
  Convert to Ah/1 -> Convert to SOC/1
  Current/1 -> Discrete-Time Integrator/1
  Convert to SOC/1 -> SOC/1

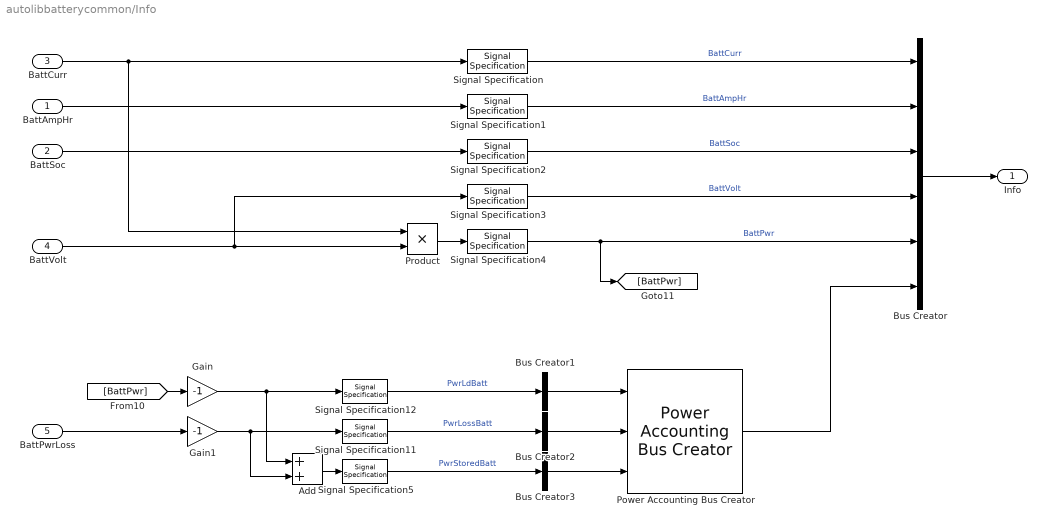
== system autolibbatterycommon/Info ==
  BattAmpHr : Inport
  BattSoc : Inport  Port=2
  BattCurr : Inport  Port=3
  BattVolt : Inport  Port=4
  BattPwrLoss : Inport  Port=5
  Add : Sum
  Bus Creator : BusCreator  Inputs=6
  Bus Creator1 : BusCreator  Inputs=1
  Bus Creator2 : BusCreator  Inputs=1
  Bus Creator3 : BusCreator  Inputs=1
  Gain : Gain  Gain=-1
  Gain1 : Gain  Gain=-1
  Power Accounting Bus Creator : autolibpowerinfoutils/Power Accounting Bus Creator  AssctBlkSelPopup=Parent reference block  RefBlkName=RefBlkName  PwrTrnsfrdCheckBox=on  PwrNotTrnsfrdCheckBox=on  PwrStoredCheckBox=on  aMode=aMode
      settings: SourceProductName=Powertrain Blockset  SourceProductBaseCode=PW
  Product : Product
  Signal Specification : SignalSpecification  Unit=A
  Signal Specification1 : SignalSpecification  Unit=A*h
  Signal Specification{4..5,11..12} (4 alike) : SignalSpecification  Unit=W
  Signal Specification2 : SignalSpecification  Unit=1
  Signal Specification3 : SignalSpecification  Unit=V
  Info : Outport  VectorParamsAs1DForOutWhenUnconnected=off
  wires:
  Signal Specification3/1 -> Bus Creator/4  "BattVolt"
  Signal Specification2/1 -> Bus Creator/3  "BattSoc"
  Signal Specification4/1 -> [BattPwr], Bus Creator/5  "BattPwr"
  Signal Specification1/1 -> Bus Creator/2  "BattAmpHr"
  Signal Specification/1 -> Bus Creator/1  "BattCurr"
  BattCurr/1 -> Signal Specification/1, Product/1
  Bus Creator/1 -> Info/1
  BattAmpHr/1 -> Signal Specification1/1
  BattSoc/1 -> Signal Specification2/1
  Product/1 -> Signal Specification4/1
  BattVolt/1 -> Signal Specification3/1, Product/2
  Signal Specification11/1 -> Bus Creator2/1  "PwrLossBatt"
  Bus Creator1/1 -> Power Accounting Bus Creator/1
  Signal Specification12/1 -> Bus Creator1/1  "PwrLdBatt"
  Bus Creator2/1 -> Power Accounting Bus Creator/2
  Bus Creator3/1 -> Power Accounting Bus Creator/3
  Signal Specification5/1 -> Bus Creator3/1  "PwrStoredBatt"
  Power Accounting Bus Creator/1 -> Bus Creator/6
  BattPwrLoss/1 -> Gain1/1
  Gain/1 -> Add/1, Signal Specification12/1
  Gain1/1 -> Add/2, Signal Specification11/1
  [BattPwr] -> Gain/1
  Add/1 -> Signal Specification5/1

== system autolibbatterycommon/Output Filter ==
  OutVoltUnfilt : Inport
  Constant1 : Constant  Value=Tc
  Constant2 : Constant  Value=Vinit
  Gain1 : Gain  Gain=1/Tc
  Integrator : Integrator  InitialConditionSource=external
  Product : Product
  Sum : Sum  Inputs=|+-
  OutVolt : Outport  VectorParamsAs1DForOutWhenUnconnected=off
  wires:
  OutVoltUnfilt/1 -> Sum/1
  Sum/1 -> Integrator/1
  Integrator/1 -> Gain1/1
  Gain1/1 -> OutVolt/1, Sum/2
  Constant2/1 -> Product/1
  Constant1/1 -> Product/2
  Product/1 -> Integrator/2

== system autolibbatterycommon/Output Passthrough ==
  OutVoltUnfilt : Inport
  OutVolt : Outport  VectorParamsAs1DForOutWhenUnconnected=off
  wires:
  OutVoltUnfilt/1 -> OutVolt/1

== system autolibbatterycommon/PE 1RC ==
  BattCurr : Inport  Unit=A
  Add : Sum  Inputs=+--
  Bus Creator : BusCreator  Inputs=1
  Em : Lookup_n-D  NumberOfTableDimensions=1  LookupTableObject=''  BreakpointsForDimension1=SOC_BP  Table=Em  ExtrapMethod=Clip  UseLastTableValue=on  InternalRulePriority=Speed  RndMeth=Simplest  InputSameDT=on
  Gain : Gain  Gain=-1
  PE RC1 : $bdroot/PE RC1  R=R1  C=C1  SOC_BP=SOC_BP  V_init=InitialCapVoltage(1)  V_upper=Vu  V_lower=Vl
  PE SOC Counter : $bdroot/PE SOC Counter  Q_init=BattCapInit  Cap=BattCap
  Product : Product
  R0 : Lookup_n-D  NumberOfTableDimensions=1  LookupTableObject=''  BreakpointsForDimension1=SOC_BP  Table=R0  ExtrapMethod=Clip  UseLastTableValue=on  InternalRulePriority=Speed  RndMeth=Simplest  InputSameDT=on
  Signal Specification : SignalSpecification  Unit=V
  Info : Outport  VectorParamsAs1DForOutWhenUnconnected=off
  BattVolt : Outport  Port=2  Unit=V  VectorParamsAs1DForOutWhenUnconnected=off
  BattSoc : Outport  Port=3  Unit=1  VectorParamsAs1DForOutWhenUnconnected=off
  wires:
  PE SOC Counter/1 -> Em/1, PE RC1/1, R0/1, BattSoc/1
  Product/1 -> Add/2
  R0/1 -> Product/1
  BattCurr/1 -> PE SOC Counter/1, PE RC1/2, Product/2
  Add/1 -> BattVolt/1
  Em/1 -> Add/1
  Bus Creator/1 -> Info/1
  PE RC1/1 -> Gain/1, Add/3
  Gain/1 -> Signal Specification/1
  Signal Specification/1 -> Bus Creator/1  "CapVolt"

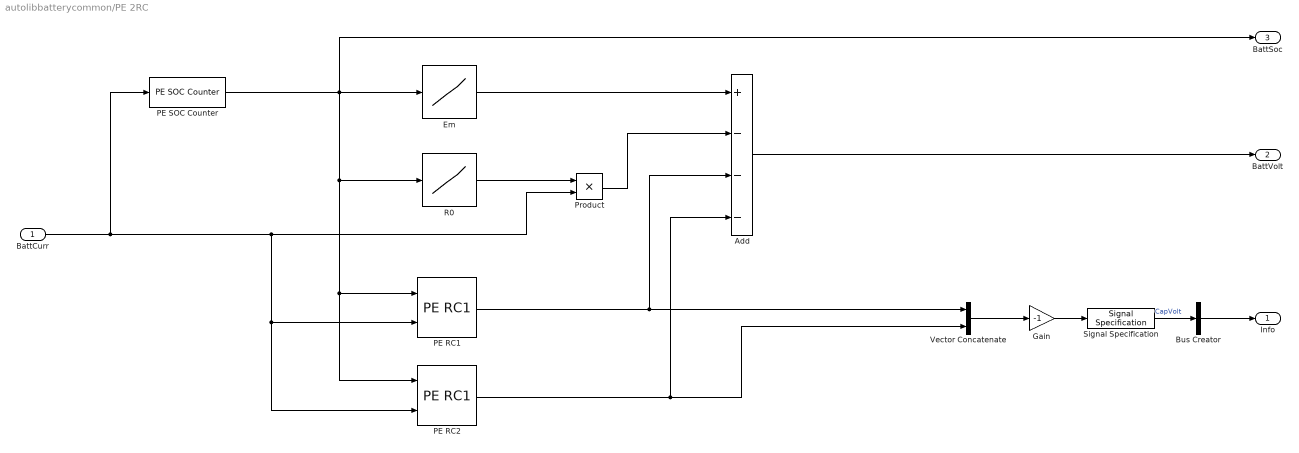
== system autolibbatterycommon/PE 2RC ==
  BattCurr : Inport  Unit=A
  Add : Sum  Inputs=+---
  Bus Creator : BusCreator  Inputs=1
  Em : Lookup_n-D  NumberOfTableDimensions=1  LookupTableObject=''  BreakpointsForDimension1=SOC_BP  Table=Em  ExtrapMethod=Clip  UseLastTableValue=on  InternalRulePriority=Speed  RndMeth=Simplest  InputSameDT=on
  Gain : Gain  Gain=-1
  PE RC1 : $bdroot/PE RC1  R=R1  C=C1  SOC_BP=SOC_BP  V_init=InitialCapVoltage(1)  V_upper=Vu  V_lower=Vl
  PE RC2 : $bdroot/PE RC1  R=R2  C=C2  SOC_BP=SOC_BP  V_init=InitialCapVoltage(2)  V_upper=Vu  V_lower=Vl
  PE SOC Counter : $bdroot/PE SOC Counter  Q_init=BattCapInit  Cap=BattCap
  Product : Product
  R0 : Lookup_n-D  NumberOfTableDimensions=1  LookupTableObject=''  BreakpointsForDimension1=SOC_BP  Table=R0  ExtrapMethod=Clip  UseLastTableValue=on  InternalRulePriority=Speed  RndMeth=Simplest  InputSameDT=on
  Signal Specification : SignalSpecification  Unit=V
  Vector Concatenate : Concatenate
  Info : Outport  VectorParamsAs1DForOutWhenUnconnected=off
  BattVolt : Outport  Port=2  Unit=V  VectorParamsAs1DForOutWhenUnconnected=off
  BattSoc : Outport  Port=3  Unit=1  VectorParamsAs1DForOutWhenUnconnected=off
  wires:
  Em/1 -> Add/1
  Add/1 -> BattVolt/1
  BattCurr/1 -> PE SOC Counter/1, PE RC2/2, PE RC1/2, Product/2
  R0/1 -> Product/1
  Product/1 -> Add/2
  PE RC1/1 -> Vector Concatenate/1, Add/3
  PE RC2/1 -> Vector Concatenate/2, Add/4
  PE SOC Counter/1 -> BattSoc/1, R0/1, PE RC2/1, PE RC1/1, Em/1
  Vector Concatenate/1 -> Gain/1
  Bus Creator/1 -> Info/1
  Gain/1 -> Signal Specification/1
  Signal Specification/1 -> Bus Creator/1  "CapVolt"

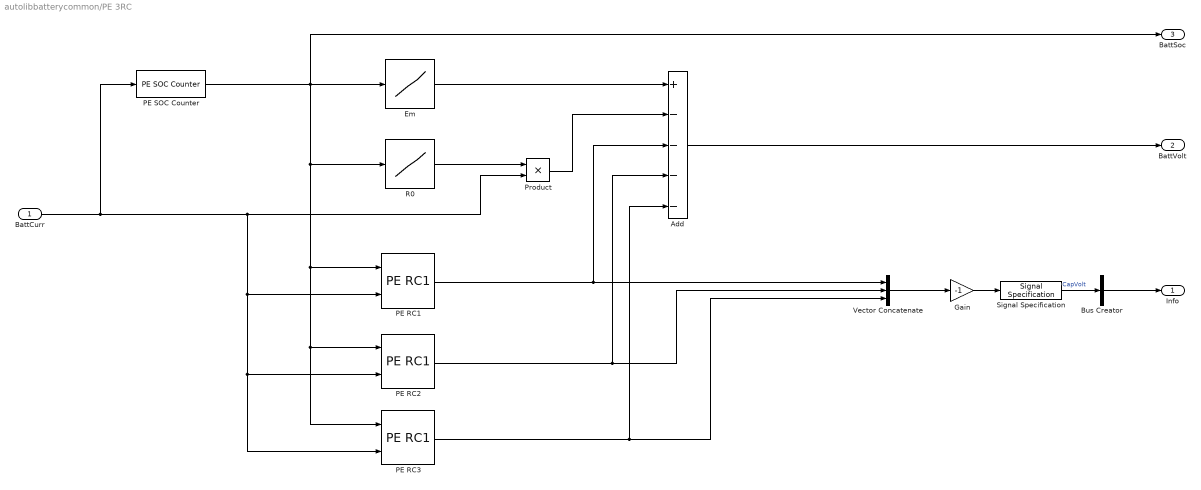
== system autolibbatterycommon/PE 3RC ==
  BattCurr : Inport  Unit=A
  Add : Sum  Inputs=+----
  Bus Creator : BusCreator  Inputs=1
  Em : Lookup_n-D  NumberOfTableDimensions=1  LookupTableObject=''  BreakpointsForDimension1=SOC_BP  Table=Em  ExtrapMethod=Clip  UseLastTableValue=on  InternalRulePriority=Speed  RndMeth=Simplest  InputSameDT=on
  Gain : Gain  Gain=-1
  PE RC1 : $bdroot/PE RC1  R=R1  C=C1  SOC_BP=SOC_BP  V_init=InitialCapVoltage(1)  V_upper=Vu  V_lower=Vl
  PE RC2 : $bdroot/PE RC1  R=R2  C=C2  SOC_BP=SOC_BP  V_init=InitialCapVoltage(2)  V_upper=Vu  V_lower=Vl
  PE RC3 : $bdroot/PE RC1  R=R3  C=C3  SOC_BP=SOC_BP  V_init=InitialCapVoltage(3)  V_upper=Inf  V_lower=-Inf
  PE SOC Counter : $bdroot/PE SOC Counter  Q_init=BattCapInit  Cap=BattCap
  Product : Product
  R0 : Lookup_n-D  NumberOfTableDimensions=1  LookupTableObject=''  BreakpointsForDimension1=SOC_BP  Table=R0  ExtrapMethod=Clip  UseLastTableValue=on  InternalRulePriority=Speed  RndMeth=Simplest  InputSameDT=on
  Signal Specification : SignalSpecification  Unit=V
  Vector Concatenate : Concatenate  NumInputs=3
  Info : Outport  VectorParamsAs1DForOutWhenUnconnected=off
  BattVolt : Outport  Port=2  Unit=V  VectorParamsAs1DForOutWhenUnconnected=off
  BattSoc : Outport  Port=3  Unit=1  VectorParamsAs1DForOutWhenUnconnected=off
  wires:
  Vector Concatenate/1 -> Gain/1
  PE SOC Counter/1 -> Em/1, PE RC1/1, PE RC3/1, PE RC2/1, R0/1, BattSoc/1
  PE RC3/1 -> Add/5, Vector Concatenate/3
  PE RC2/1 -> Vector Concatenate/2, Add/4
  PE RC1/1 -> Vector Concatenate/1, Add/3
  Product/1 -> Add/2
  R0/1 -> Product/1
  BattCurr/1 -> PE SOC Counter/1, Product/2, PE RC1/2, PE RC3/2, PE RC2/2
  Add/1 -> BattVolt/1
  Em/1 -> Add/1
  Bus Creator/1 -> Info/1
  Gain/1 -> Signal Specification/1
  Signal Specification/1 -> Bus Creator/1  "CapVolt"

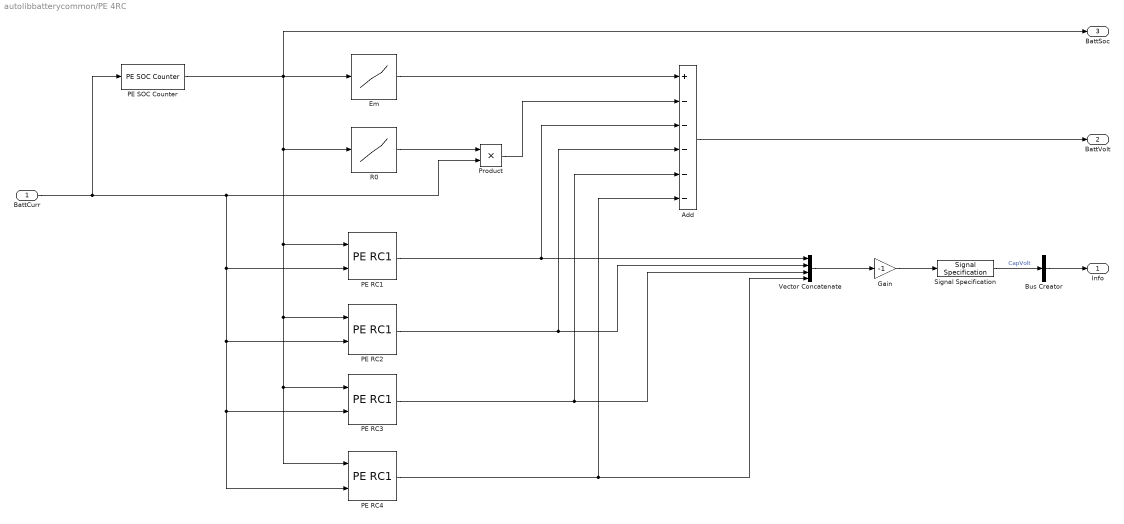
== system autolibbatterycommon/PE 4RC ==
  BattCurr : Inport  Unit=A
  Add : Sum  Inputs=+-----
  Bus Creator : BusCreator  Inputs=1
  Em : Lookup_n-D  NumberOfTableDimensions=1  LookupTableObject=''  BreakpointsForDimension1=SOC_BP  Table=Em  ExtrapMethod=Clip  UseLastTableValue=on  InternalRulePriority=Speed  RndMeth=Simplest  InputSameDT=on
  Gain : Gain  Gain=-1
  PE RC1 : $bdroot/PE RC1  R=R1  C=C1  SOC_BP=SOC_BP  V_init=InitialCapVoltage(1)  V_upper=Vu  V_lower=Vl
  PE RC2 : $bdroot/PE RC1  R=R2  C=C2  SOC_BP=SOC_BP  V_init=InitialCapVoltage(2)  V_upper=Vu  V_lower=Vl
  PE RC3 : $bdroot/PE RC1  R=R3  C=C3  SOC_BP=SOC_BP  V_init=InitialCapVoltage(3)  V_upper=Inf  V_lower=-Inf
  PE RC4 : $bdroot/PE RC1  R=R4  C=C4  SOC_BP=SOC_BP  V_init=InitialCapVoltage(4)  V_upper=Vu  V_lower=Vl
  PE SOC Counter : $bdroot/PE SOC Counter  Q_init=BattCapInit  Cap=BattCap
  Product : Product
  R0 : Lookup_n-D  NumberOfTableDimensions=1  LookupTableObject=''  BreakpointsForDimension1=SOC_BP  Table=R0  ExtrapMethod=Clip  UseLastTableValue=on  InternalRulePriority=Speed  RndMeth=Simplest  InputSameDT=on
  Signal Specification : SignalSpecification  Unit=V
  Vector Concatenate : Concatenate  NumInputs=4
  Info : Outport  VectorParamsAs1DForOutWhenUnconnected=off
  BattVolt : Outport  Port=2  Unit=V  VectorParamsAs1DForOutWhenUnconnected=off
  BattSoc : Outport  Port=3  Unit=1  VectorParamsAs1DForOutWhenUnconnected=off
  wires:
  PE RC4/1 -> Vector Concatenate/4, Add/6
  Em/1 -> Add/1
  Add/1 -> BattVolt/1
  BattCurr/1 -> PE SOC Counter/1, PE RC1/2, PE RC2/2, PE RC4/2, PE RC3/2, Product/2
  R0/1 -> Product/1
  Product/1 -> Add/2
  PE RC1/1 -> Vector Concatenate/1, Add/3
  PE RC2/1 -> Vector Concatenate/2, Add/4
  PE RC3/1 -> Vector Concatenate/3, Add/5
  PE SOC Counter/1 -> BattSoc/1, R0/1, PE RC1/1, PE RC2/1, PE RC4/1, PE RC3/1, Em/1
  Vector Concatenate/1 -> Gain/1
  Bus Creator/1 -> Info/1
  Gain/1 -> Signal Specification/1
  Signal Specification/1 -> Bus Creator/1  "CapVolt"

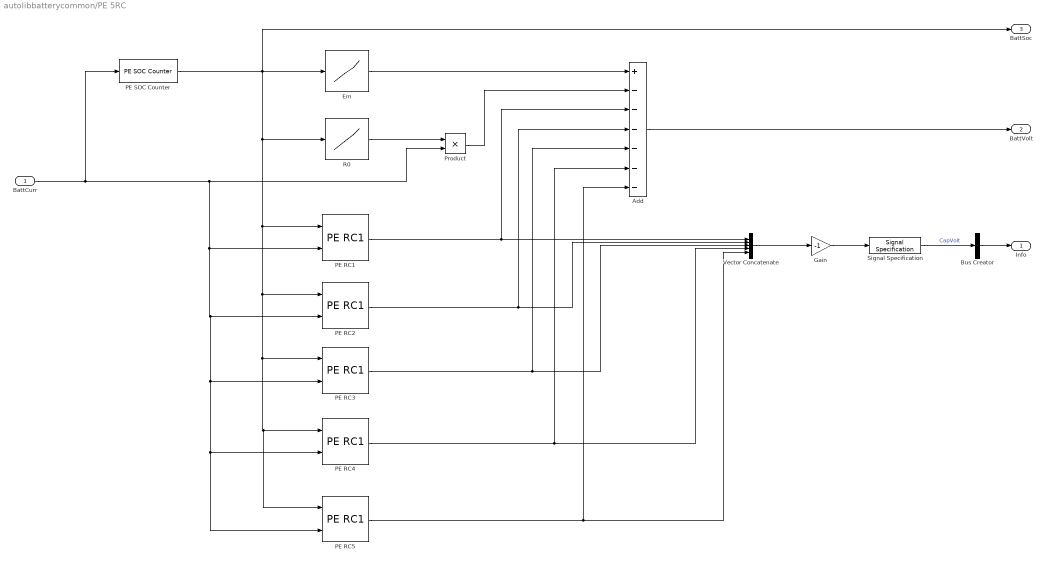
== system autolibbatterycommon/PE 5RC ==
  BattCurr : Inport  Unit=A
  Add : Sum  Inputs=+------
  Bus Creator : BusCreator  Inputs=1
  Em : Lookup_n-D  NumberOfTableDimensions=1  LookupTableObject=''  BreakpointsForDimension1=SOC_BP  Table=Em  ExtrapMethod=Clip  UseLastTableValue=on  InternalRulePriority=Speed  RndMeth=Simplest  InputSameDT=on
  Gain : Gain  Gain=-1
  PE RC1 : $bdroot/PE RC1  R=R1  C=C1  SOC_BP=SOC_BP  V_init=InitialCapVoltage(1)  V_upper=Vu  V_lower=Vl
  PE RC2 : $bdroot/PE RC1  R=R2  C=C2  SOC_BP=SOC_BP  V_init=InitialCapVoltage(2)  V_upper=Vu  V_lower=Vl
  PE RC3 : $bdroot/PE RC1  R=R3  C=C3  SOC_BP=SOC_BP  V_init=InitialCapVoltage(3)  V_upper=Vu  V_lower=Vl
  PE RC4 : $bdroot/PE RC1  R=R4  C=C4  SOC_BP=SOC_BP  V_init=InitialCapVoltage(4)  V_upper=Vu  V_lower=Vl
  PE RC5 : $bdroot/PE RC1  R=R5  C=C5  SOC_BP=SOC_BP  V_init=InitialCapVoltage(5)  V_upper=Vu  V_lower=Vl
  PE SOC Counter : $bdroot/PE SOC Counter  Q_init=BattCapInit  Cap=BattCap
  Product : Product
  R0 : Lookup_n-D  NumberOfTableDimensions=1  LookupTableObject=''  BreakpointsForDimension1=SOC_BP  Table=R0  ExtrapMethod=Clip  UseLastTableValue=on  InternalRulePriority=Speed  RndMeth=Simplest  InputSameDT=on
  Signal Specification : SignalSpecification  Unit=V
  Vector Concatenate : Concatenate  NumInputs=5
  Info : Outport  VectorParamsAs1DForOutWhenUnconnected=off
  BattVolt : Outport  Port=2  Unit=V  VectorParamsAs1DForOutWhenUnconnected=off
  BattSoc : Outport  Port=3  Unit=1  VectorParamsAs1DForOutWhenUnconnected=off
  wires:
  PE RC5/1 -> Vector Concatenate/5, Add/7
  Vector Concatenate/1 -> Gain/1
  PE SOC Counter/1 -> PE RC1/1, PE RC2/1, PE RC3/1, PE RC5/1, PE RC4/1, R0/1, Em/1, BattSoc/1
  PE RC3/1 -> Vector Concatenate/3, Add/5
  PE RC2/1 -> Vector Concatenate/2, Add/4
  PE RC1/1 -> Vector Concatenate/1, Add/3
  Product/1 -> Add/2
  R0/1 -> Product/1
  BattCurr/1 -> PE SOC Counter/1, Product/2, PE RC1/2, PE RC2/2, PE RC3/2, PE RC5/2, PE RC4/2
  Add/1 -> BattVolt/1
  Em/1 -> Add/1
  PE RC4/1 -> Vector Concatenate/4, Add/6
  Bus Creator/1 -> Info/1
  Gain/1 -> Signal Specification/1
  Signal Specification/1 -> Bus Creator/1  "CapVolt"

== system autolibbatterycommon/PE RC1 ==
  SOC : Inport
  I : Inport  Port=2
  1-D Lookup Table2 : Lookup_n-D  NumberOfTableDimensions=1  LookupTableObject=''  BreakpointsForDimension1=SOC_BP  BreakpointsForDimension2=Current_BP  Table=R  ExtrapMethod=Clip  UseLastTableValue=on  InternalRulePriority=Speed  RndMeth=Simplest  InputSameDT=on
  1-D Lookup Table3 : Lookup_n-D  NumberOfTableDimensions=1  LookupTableObject=''  BreakpointsForDimension1=SOC_BP  BreakpointsForDimension2=Current_BP  Table=C  ExtrapMethod=Clip  UseLastTableValue=on  InternalRulePriority=Speed  RndMeth=Simplest  InputSameDT=on
  Divide1 : Product  Inputs=*/
  Divide2 : Product  Inputs=*//
  Integrator : Integrator  InitialCondition=V_init  LimitOutput=on  UpperSaturationLimit=V_upper  LowerSaturationLimit=V_lower
  Subtract : Sum  Inputs=+-
  V : Outport  VectorParamsAs1DForOutWhenUnconnected=off
  wires:
  Divide1/1 -> Subtract/1
  Subtract/1 -> Integrator/1
  Integrator/1 -> Divide2/1, V/1
  SOC/1 -> 1-D Lookup Table2/1, 1-D Lookup Table3/1
  1-D Lookup Table2/1 -> [R]
  I/1 -> Divide1/1
  [C] -> Divide1/2
  Divide2/1 -> Subtract/2
  [R] -> Divide2/2
  [C] -> Divide2/3
  1-D Lookup Table3/1 -> [C]

== system autolibbatterycommon/PE SOC Counter ==
  Current : Inport
  Charge accumulator : Integrator  InitialCondition=Q_init  LimitOutput=on  LowerSaturationLimit=0
  Convert to Ah : Gain  Gain=-1/3600
  Convert to SOC : Gain  Gain=1/Cap
  SOC : Outport  VectorParamsAs1DForOutWhenUnconnected=off
  wires:
  Charge accumulator/1 -> Convert to SOC/1
  Current/1 -> Convert to Ah/1
  Convert to SOC/1 -> SOC/1
  Convert to Ah/1 -> Charge accumulator/1

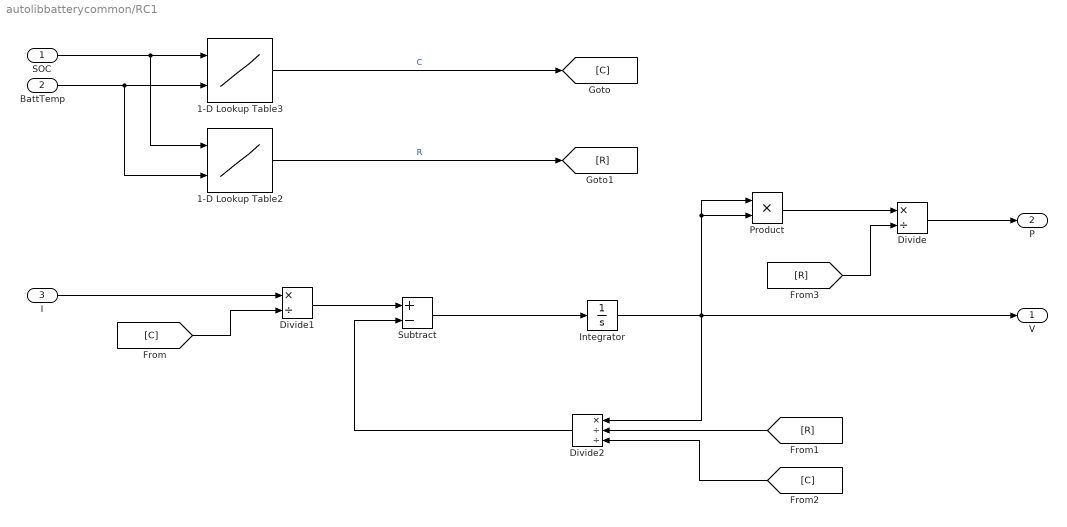
== system autolibbatterycommon/RC1 ==
  SOC : Inport
  BattTemp : Inport  Port=2
  I : Inport  Port=3
  1-D Lookup Table2 : Lookup_n-D  LookupTableObject=''  BreakpointsForDimension1=SOC_BP  BreakpointsForDimension2=Temperature_BP  Table=R  ExtrapMethod=Clip  UseLastTableValue=on  InternalRulePriority=Speed  RndMeth=Simplest  InputSameDT=on
  1-D Lookup Table3 : Lookup_n-D  LookupTableObject=''  BreakpointsForDimension1=SOC_BP  BreakpointsForDimension2=Temperature_BP  Table=C  ExtrapMethod=Clip  UseLastTableValue=on  InternalRulePriority=Speed  RndMeth=Simplest  InputSameDT=on
  Divide : Product  Inputs=*/
  Divide1 : Product  Inputs=*/
  Divide2 : Product  Inputs=*//
  Integrator : Integrator  InitialCondition=V_init  LimitOutput=on  UpperSaturationLimit=V_upper  LowerSaturationLimit=V_lower
  Product : Product
  Subtract : Sum  Inputs=+-
  V : Outport  VectorParamsAs1DForOutWhenUnconnected=off
  P : Outport  Port=2  VectorParamsAs1DForOutWhenUnconnected=off
  wires:
  [C] -> Divide2/3
  [R] -> Divide2/2
  Divide2/1 -> Subtract/2
  [C] -> Divide1/2
  I/1 -> Divide1/1
  1-D Lookup Table3/1 -> [C]  "C"
  1-D Lookup Table2/1 -> [R]  "R"
  SOC/1 -> 1-D Lookup Table2/1, 1-D Lookup Table3/1
  Integrator/1 -> Product/2, Product/1, V/1, Divide2/1
  Subtract/1 -> Integrator/1
  Divide1/1 -> Subtract/1
  BattTemp/1 -> 1-D Lookup Table2/2, 1-D Lookup Table3/2
  Product/1 -> Divide/1
  Divide/1 -> P/1
  [R] -> Divide/2

== system autolibbatterycommon/SOC Counter ==
  CapInit : Inport
  Current : Inport  Port=2
  Temp : Inport  Port=3
  Capacity : Lookup_n-D  NumberOfTableDimensions=1  BreakpointsForDimension1=Temp_BP  Table=Cap_LUT  ExtrapMethod=Clip  UseLastTableValue=on  InternalRulePriority=Speed  RndMeth=Simplest  InputSameDT=on
  Charge accumulator : Integrator  InitialConditionSource=external  InitialCondition=Q_init*3600  LimitOutput=on  LowerSaturationLimit=0
  Convert to Ah : Gain  Gain=-1/3600
  Divide1 : Product  Inputs=*/
  SOC : Outport  VectorParamsAs1DForOutWhenUnconnected=off
  LdAmpHr : Outport  Port=2  VectorParamsAs1DForOutWhenUnconnected=off
  wires:
  Current/1 -> Convert to Ah/1
  Temp/1 -> Capacity/1
  Capacity/1 -> Divide1/2
  CapInit/1 -> Charge accumulator/2
  Charge accumulator/1 -> LdAmpHr/1, Divide1/1
  Divide1/1 -> SOC/1
  Convert to Ah/1 -> Charge accumulator/1

== system autolibbatterycommon/nRC_Battery_Core ==
  note: 1) Add Subsystem or Model blocks as valid variant choices.
      | 2) You cannot connect blocks at this level. At simulation, connectivity is automatically
      | determined, based on the active variant and port name matching.
  Current : Inport
  1RC : Subsystem  VariantControl=1
  2RC : Subsystem  VariantControl=2
  3RC : Subsystem  VariantControl=3
  4RC : Subsystem  VariantControl=4
  5RC : Subsystem  VariantControl=5
  SOC : Outport  VectorParamsAs1DForOutWhenUnconnected=off
  Voltage : Outport  Port=2  VectorParamsAs1DForOutWhenUnconnected=off

== system autolibbatterycommon/1RC/Power ==
  R0 : Inport
  BattAmp : Inport  Port=2
  P1 : Inport  Port=3
  Add : Sum
  Product1 : Product  Inputs=3
  BattPwrLoss : Outport  VectorParamsAs1DForOutWhenUnconnected=off
  wires:
  R0/1 -> Product1/1
  Product1/1 -> Add/1
  Add/1 -> BattPwrLoss/1
  P1/1 -> Add/2
  BattAmp/1 -> Product1/2, Product1/3

== system autolibbatterycommon/1RC/Voltage ==
  Em : Inport
  R0 : Inport  Port=2
  BattAmp : Inport  Port=3
  RC1 : Inport  Port=4
  Add : Sum  Inputs=+--
  Product : Product
  BattVolt : Outport  VectorParamsAs1DForOutWhenUnconnected=off
  wires:
  BattAmp/1 -> Product/2
  Product/1 -> Add/2
  RC1/1 -> Add/3
  R0/1 -> Product/1
  Em/1 -> Add/1
  Add/1 -> BattVolt/1

== system autolibbatterycommon/2RC/Power ==
  R0 : Inport
  BattAmp : Inport  Port=2
  P1 : Inport  Port=3
  P2 : Inport  Port=4
  Add : Sum  Inputs=+++
  Product1 : Product  Inputs=3
  BattPwrLoss : Outport  VectorParamsAs1DForOutWhenUnconnected=off
  wires:
  R0/1 -> Product1/1
  Product1/1 -> Add/1
  Add/1 -> BattPwrLoss/1
  P1/1 -> Add/2
  BattAmp/1 -> Product1/2, Product1/3
  P2/1 -> Add/3

== system autolibbatterycommon/2RC/Voltage ==
  Em : Inport
  R0 : Inport  Port=2
  BattAmp : Inport  Port=3
  RC1 : Inport  Port=4
  RC2 : Inport  Port=5
  Add : Sum  Inputs=+---
  Product : Product
  BattVolt : Outport  VectorParamsAs1DForOutWhenUnconnected=off
  wires:
  Product/1 -> Add/2
  R0/1 -> Product/1
  RC1/1 -> Add/3
  Em/1 -> Add/1
  Add/1 -> BattVolt/1
  RC2/1 -> Add/4
  BattAmp/1 -> Product/2

== system autolibbatterycommon/3RC/Power ==
  R0 : Inport
  BattAmp : Inport  Port=2
  P1 : Inport  Port=3
  P2 : Inport  Port=4
  P3 : Inport  Port=5
  Add : Sum  Inputs=++++
  Product1 : Product  Inputs=3
  BattPwrLoss : Outport  VectorParamsAs1DForOutWhenUnconnected=off
  wires:
  R0/1 -> Product1/1
  Product1/1 -> Add/1
  Add/1 -> BattPwrLoss/1
  P1/1 -> Add/2
  BattAmp/1 -> Product1/2, Product1/3
  P2/1 -> Add/3
  P3/1 -> Add/4

== system autolibbatterycommon/3RC/Voltage ==
  Em : Inport
  R0 : Inport  Port=2
  BattAmp : Inport  Port=3
  RC1 : Inport  Port=4
  RC2 : Inport  Port=5
  RC3 : Inport  Port=6
  Add : Sum  Inputs=+----
  Product : Product
  BattVolt : Outport  VectorParamsAs1DForOutWhenUnconnected=off
  wires:
  BattAmp/1 -> Product/2
  RC3/1 -> Add/5
  Add/1 -> BattVolt/1
  R0/1 -> Product/1
  Product/1 -> Add/2
  RC1/1 -> Add/3
  Em/1 -> Add/1
  RC2/1 -> Add/4

== system autolibbatterycommon/4RC/Power ==
  R0 : Inport
  BattAmp : Inport  Port=2
  P1 : Inport  Port=3
  P2 : Inport  Port=4
  P3 : Inport  Port=5
  P4 : Inport  Port=6
  Add : Sum  Inputs=+++++
  Product1 : Product  Inputs=3
  BattPwrLoss : Outport  VectorParamsAs1DForOutWhenUnconnected=off
  wires:
  R0/1 -> Product1/1
  Product1/1 -> Add/1
  Add/1 -> BattPwrLoss/1
  P1/1 -> Add/2
  BattAmp/1 -> Product1/2, Product1/3
  P2/1 -> Add/3
  P3/1 -> Add/4
  P4/1 -> Add/5

== system autolibbatterycommon/4RC/Voltage ==
  Em : Inport
  R0 : Inport  Port=2
  BattAmp : Inport  Port=3
  RC1 : Inport  Port=4
  RC2 : Inport  Port=5
  RC3 : Inport  Port=6
  RC4 : Inport  Port=7
  Add : Sum  Inputs=+-----
  Product : Product
  BattVolt : Outport  VectorParamsAs1DForOutWhenUnconnected=off
  wires:
  Em/1 -> Add/1
  Add/1 -> BattVolt/1
  RC3/1 -> Add/5
  RC1/1 -> Add/3
  Product/1 -> Add/2
  R0/1 -> Product/1
  RC4/1 -> Add/6
  RC2/1 -> Add/4
  BattAmp/1 -> Product/2

== system autolibbatterycommon/5RC/Power ==
  R0 : Inport
  BattAmp : Inport  Port=2
  P1 : Inport  Port=3
  P2 : Inport  Port=4
  P3 : Inport  Port=5
  P4 : Inport  Port=6
  P5 : Inport  Port=7
  Add : Sum  Inputs=++++++
  Product1 : Product  Inputs=3
  BattPwrLoss : Outport  VectorParamsAs1DForOutWhenUnconnected=off
  wires:
  R0/1 -> Product1/1
  Product1/1 -> Add/1
  Add/1 -> BattPwrLoss/1
  P1/1 -> Add/2
  BattAmp/1 -> Product1/2, Product1/3
  P2/1 -> Add/3
  P3/1 -> Add/4
  P4/1 -> Add/5
  P5/1 -> Add/6
